simulink model "carModel"  (R2021a)
settings: Solver=ode15s  StartTime=0.0  StopTime=50  MaxStep=0.5  RelTol=1e-3
values from neighbouring files (symbols this model uses):
  initialFuel = 100    [data.m]
  maxEngineTemp = 240    [data.m]
  maxEngineTorque = 80    [data.m]
  maxMotorTemp = 135    [data.m]
  maxMotorTorque = 80    [data.m]
  maxRegenTorque = 80    [data.m]
  motorVoltage = 140    [data.m]
undefined symbols (not defined in the file or in its folder): b, k, Lock, N, sigbuilder_block, Temp_bpts, up
libraries: autolibsharedcoupling x7, autolibshared x7, autolibpowerinfoutils x4, autolibshareddiff x3, autolibhevctrlrcommon x2, autolibtrqconv x2, autolibutils x2, autolibtransamt x1, autolibsharedtransfixedgear x1, autolibdcdc x1, autolibdatasheetbattery x1, autolibmappedmotor x1
(part 1 of 6)
settings Model: EnablePacing=on  PacingRate=10  Creator=peter  LastModifiedBy=peter
settings DebuggingCC: SFMachineParentedDataDiag=warning

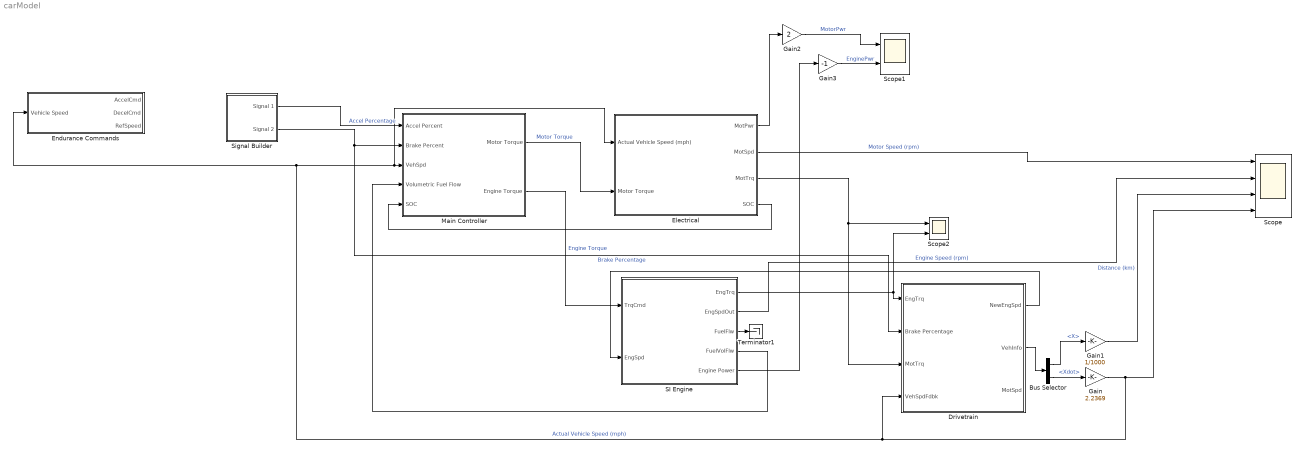
== system carModel ==
  Bus Selector : BusSelector  OutputSignals=InertFrm.Cg.Disp.X,InertFrm.Cg.Vel.Xdot
  Drivetrain : Subsystem
  Electrical : Subsystem
  Endurance Commands : Subsystem
  Gain : Gain  Gain=2.2369
  Gain1 : Gain  Gain=1/1000
  Gain2 : Gain  Gain=2
  Gain3 : Gain  Gain=-1
  Main Controller : Subsystem
  SI Engine : Subsystem
  Scope : Scope  NumInputPorts=4
  Scope1 : Scope  NumInputPorts=2
  Scope2 : Scope  NumInputPorts=2
  Signal Builder : Subsystem  Tag=STV Subsys  LoadFcn=sigbuilder_block('load');  StartFcn=sigbuilder_block('start');  StopFcn=sigbuilder_block('stop');  ClipboardFcn=sigbuilder_block('clipboard');  mask(Sigbuilder block){tuvar=[0:10]}
      mask help: Simulink:masks:SigbuilderBlock_MD
      mask init:
      | if ~strcmp(get_param(bdroot(gcbh),'SimulationStatus'),'stopped') tuvar = sigbuilder_block('maskInit'); end
      settings: CopyFcn=sigbuilder_block('copy');  DeleteFcn=sigbuilder_block('delete');  ModelCloseFcn=sigbuilder_block('modelClose');  PreSaveFcn=sigbuilder_block('preSave');  PauseFcn=sigbuilder_block('pause');  ContinueFcn=sigbuilder_block('continue');  NameChangeFcn=sigbuilder_block('namechange');  OpenFcn=sigbuilder_block('open',[1896 -18 550.8 400.2 ]);  CloseFcn=sigbuilder_block('close');
      mask Display: plot(0, 0, 100, 100,[2, 2, 32, 32, 2], [68, 8, 8, 68, 68],[32, 2], [38, 38], [32, 19, 2],[53, 60, 44], [32, 17, 17, 2],[16, 16, 31, 31]);txt = getActiveGroup(gcbh);text(2, 100, txt,'verticalAlignment', 'top');
  Terminator1 : Terminator
  wires:
  Electrical/4(SOC) -> Main Controller/5(SOC)
  Main Controller/1(Motor Torque) -> Electrical/2(Motor Torque)  "Motor Torque"
  Main Controller/2(Engine Torque) -> SI Engine/1(TrqCmd)  "Engine Torque"
  Drivetrain/1(NewEngSpd) -> SI Engine/2(EngSpd)
  SI Engine/3(FuelFlw) -> Terminator1/1
  SI Engine/4(FuelVolFlw) -> Main Controller/4(Volumetric Fuel Flow)
  SI Engine/1(EngTrq) -> Scope2/2, Drivetrain/1(EngTrq)
  Electrical/3(MotTrq) -> Drivetrain/3(MotTrq), Scope2/1
  Electrical/2(MotSpd) -> Scope/1  "Motor Speed (rpm)"
  Drivetrain/2(VehInfo) -> Bus Selector/1
  Bus Selector/1 -> Gain1/1  "<X>"
  Bus Selector/2 -> Gain/1  "<Xdot>"
  Gain/1 -> Scope/4, Drivetrain/4(VehSpdFdbk), Endurance Commands/1(Vehicle Speed), Electrical/1(Actual Vehicle Speed (mph)), Main Controller/3(VehSpd)  "Actual Vehicle Speed (mph)"
  Gain1/1 -> Scope/3  "Distance (km)"
  SI Engine/5(Engine Power) -> Gain3/1
  Electrical/1(MotPwr) -> Gain2/1
  Gain2/1 -> Scope1/1  "MotorPwr"
  Gain3/1 -> Scope1/2  "EnginePwr"
  SI Engine/2(EngSpdOut) -> Scope/2  "Engine Speed (rpm)"
  Signal Builder/1(Signal 1) -> Main Controller/1(Accel Percent)  "Accel Percentage"
  Signal Builder/2(Signal 2) -> Drivetrain/2(Brake Percentage), Main Controller/2(Brake Percent)  "Brake Percentage"

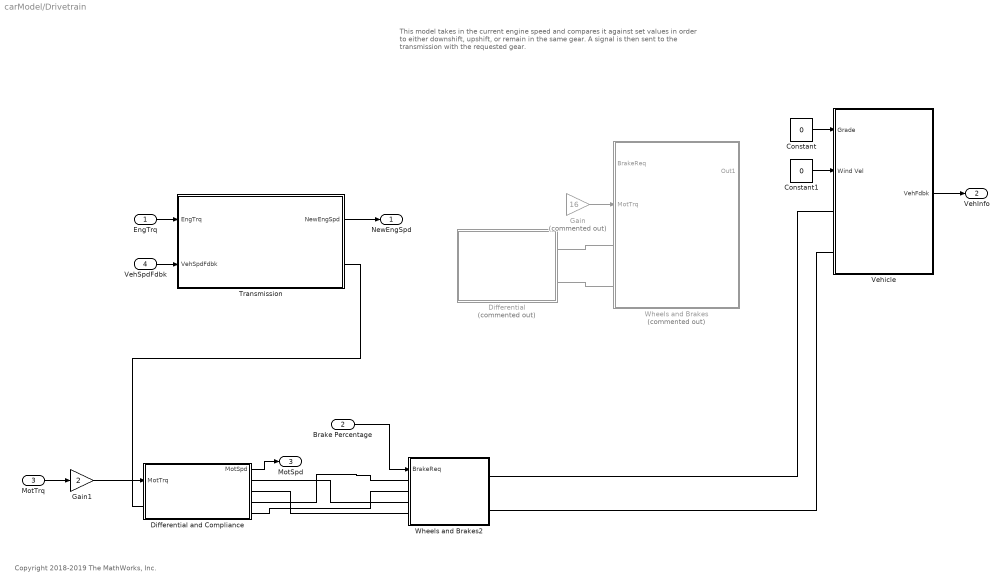
== system carModel/Drivetrain ==
  note: This model takes in the current engine speed and compares it against set values in order to either downshift, upshift, or remain in the same gear. A signal is then sent to the transmission with the requested gear.
  note: Copyright 2018-2019 The MathWorks, Inc.
  EngTrq : Inport
  Brake Percentage : Inport  Port=2
  MotTrq : Inport  Port=3
  VehSpdFdbk : Inport  Port=4
  Constant : Constant  Value=0
  Constant1 : Constant  Value=0
  Differential : Subsystem  Commented=on
  Differential and Compliance : Subsystem  VariantControl=2
  Gain : Gain  Commented=on  Gain=16
  Gain1 : Gain  Gain=2
  Transmission : Subsystem
  Vehicle : Subsystem
  Wheels and Brakes : Subsystem  Commented=on  VariantControl=0
  Wheels and Brakes2 : Subsystem  VariantControl=0
  NewEngSpd : Outport
  VehInfo : Outport  Port=2
  MotSpd : Outport  Port=3  VectorParamsAs1DForOutWhenUnconnected=off  BusOutputAsStruct=on
  wires:
  Constant/1 -> Vehicle/1(Grade)
  Constant1/1 -> Vehicle/2(Wind Vel)
  VehSpdFdbk/1 -> Transmission/2(VehSpdFdbk)
  Transmission/1(NewEngSpd) -> NewEngSpd/1
  Vehicle/1(VehFdbk) -> VehInfo/1
  Gain/1 -> Wheels and Brakes/2(MotTrq)
  EngTrq/1 -> Transmission/1(EngTrq)
  Differential and Compliance/1(MotSpd) -> MotSpd/1
  MotTrq/1 -> Gain1/1
  Brake Percentage/1 -> Wheels and Brakes2/1(BrakeReq)
  Gain1/1 -> Differential and Compliance/1(MotTrq)
  connections:
  Differential/RConn1 -- Wheels and Brakes/LConn1
  Differential/RConn2 -- Wheels and Brakes/LConn2
  Wheels and Brakes2/RConn2 -- Vehicle/LConn2
  Wheels and Brakes2/RConn1 -- Vehicle/LConn1
  Transmission/RConn1 -- Differential and Compliance/LConn1
  Differential and Compliance/RConn1 -- Wheels and Brakes2/LConn3
  Differential and Compliance/RConn2 -- Wheels and Brakes2/LConn4
  Differential and Compliance/RConn3 -- Wheels and Brakes2/LConn1
  Differential and Compliance/RConn4 -- Wheels and Brakes2/LConn2

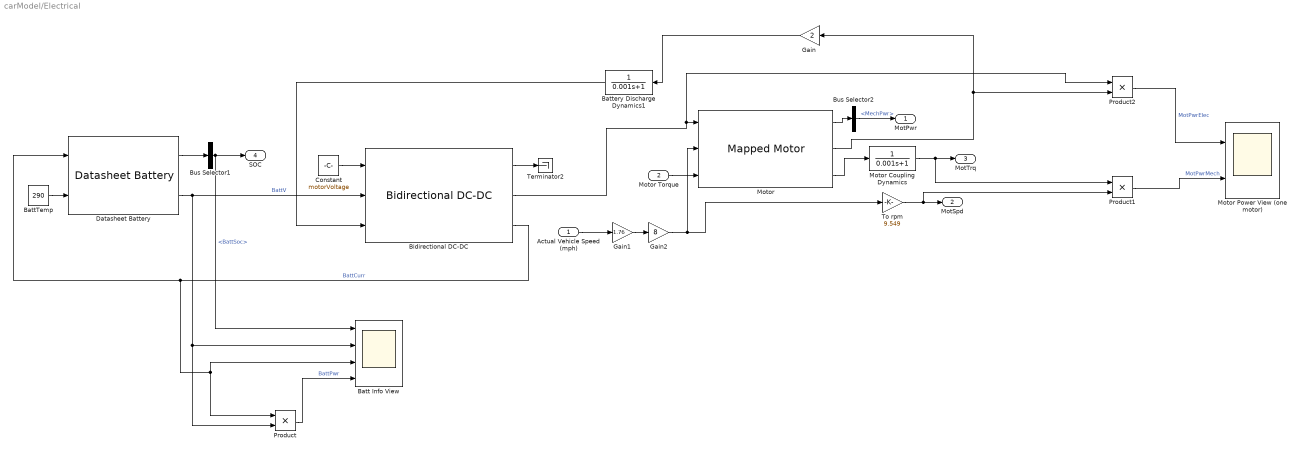
== system carModel/Electrical ==
  Actual Vehicle Speed (mph) : Inport
  Motor Torque : Inport  Port=2
  Batt Info View : Scope  NumInputPorts=4
  BattTemp : Constant  Value=290
  Battery Discharge Dynamics1 : TransferFcn  Denominator=[0.001 1]
  Bidirectional DC-DC : autolibdcdc/Bidirectional DC-DC  Tc=1/1000  Vinit=motorVoltage  Plimit=30000  param_loss=Single efficiency measurement  eff=98  v_loss_bp=[0 200 400 600 800 1000]  i_loss_bp=[0 25 50 75 100]  losses_table=[100 100 100 100 100;100 150 200 250 300;100 200 300 400 500;100 250 400 550 700;100 300 500 700 900;100 350 600 850 1100]  v_eff_bp=[200 400 600 800 1000]  i_eff_bp=[25 50 75 100]  efficiency_table=[96.2 98.1 98.7 99;98.1 99 99.4 99.5;98.7 99.4 99.6 99.7;99 99.5 99.7 99.8;99.2 99.6 99.7 99.8]  x_v_bp=[-1000 -800 -600 -400 -200 200 400 600 800 1000]  x_i_bp=[-100 -75 -50 -25 25 50 75 100]  x_losses_mat=[200.400801603196 225.67703109328 200.803212851408 201.612903225806 199.999999999997 200 225 200;160.320641282556 180.541624874624 201.005025125625 202.020202020203 200 200 180 160;180.541624874624 180.722891566267 181.086519114686 197.568389057748 194.999999999999 179.999999999997 180 180;201.005025125625 181.086519114686 202.020202020203 193.67991845056 190 200 179.999999999997 200;202.020202020203 197.568389057748 193.67991845056 197.505197505197 190 190 194.999999999999 200;200 194.999999999999 190 190 197.505197505197 193.67991845056 197.568389057748 202.020202020203;200 179.999999999997 200 190 193.67991845056 202.020202020203 181.086519114686 201.005025125625;180 180 179.999999999997 194.999999999999 197.568389057748 181.086519114686 180.722891566267 180.541624874624;160 180 200 200 202.020202020203 201.005025125625 180.541624874624 160.320641282556;200 225 200 199.999999999997 201.612903225806 200.803212851408 225.67703109328 200.400801603196]  RefBlkName='autolibdcdc/Bidirectional DC-DC'
      settings: SourceProductBaseCode=PW
  Bus Selector1 : BusSelector  OutputSignals=BattSoc
  Bus Selector2 : BusSelector  OutputSignals=MechPwr
  Constant : Constant  Value=motorVoltage
  Datasheet Battery : autolibdatasheetbattery/Datasheet Battery  CapacityCtrl=Parameter  OutputVlt=Filtered  BattChargeMax=2.5  Em=[2.8 3.228 3.284 3.361 3.408 3.427 3.472 3.477 3.493 3.504 3.516 3.528 3.537 3.545 3.555 3.561 3.566 3.576 3.587 3.589 3.594 3.6 3.608 3.61 3.616 3.619 3.626 3.632 3.637 3.64 3.645 3.646 3.652 3.655 3.658 3.661 3.664 3.668 3.673 3.678 3.68 3.681 3.686 3.692 3.699 3.702 3.705 3.71 3.717 3.723 3.728 3.733 3.735 3.742 3.749 3.755 3.761 3.768 3.773 3.78 3.791 3.798 3.798 3.814 3.818 3.825 3.841 3.846 3.855 3.863 3.877 3.885 3.894 3.907 3.919 3.926 3.935 3.944 3.954 3.964 3.974 3.988 3.998 4.014 4.029 4.034 4.047 4.065 4.074 4.086 4.097 4.131 4.126 4.138 4.15 4.18 4.174 4.187 4.207 4.231 4.221]  CapLUTBp=[0 0.01 0.02 0.03 0.04 0.05 0.06 0.07 0.08 0.09 0.1 0.11 0.12 0.13 0.14 0.15 0.16 0.17 0.18 0.19 0.2 0.21 0.22 0.23 0.24 0.25 0.26 0.27 0.28 0.29 0.3 0.31 0.32 0.33 0.34 0.35 0.36 0.37 0.38 0.39 0.4 0.41 0.42 0.43 0.44 0.45 0.46 0.47 0.48 0.49 0.5 0.51 0.52 0.53 0.54 0.55 0.56 0.57 0.58 0.59 0.6 0.61 0.62 0.63 0.64 0.65 0.66 0.67 0.68 0.69 0.7 0.71 0.72 0.73 0.74 0.75 0.76 0.77 0.78 0.79 0.8 0.81 0.82 0.83 0.84 0.85 0.86 0.87 0.88 0.89 0.9 0.91 0.92 0.93 0.94 0.95 0.96 0.97 0.98 0.99 1]  RInt=[0.008846 0.009319 0.009027 0.00847 0.01032 0.01314;0.006389 0.006554 0.005553 0.005525 0.006043 0.007805;0.004364 0.004101 0.00406 0.003452 0.003846 0.004517;0.002031 0.002563 0.002532 0.00246 0.002716 0.003047;0.001443 0.001825 0.001795 0.001778 0.001924 0.002234;0.0005603 0.0007192 0.0006887 0.0007557 0.0007355 0.001014;0.001028 0.001338 0.001 0.001536 0.001546 0.002789]  BattTempBp=[243.1 253.1 263.1 273.1 283.1 298.1 313.1]  CapSOCBp=[0 0.2 0.4 0.6 0.8 1]  Ns=32  Np=9  BattCapInit=2.5  Tc=1/1000  Vinit=4.221  RefBlkName='autolibdatasheetbattery/Datasheet Battery'
      settings: SourceProductBaseCode=PW
  Gain : Gain  Gain=2
  Gain1 : Gain  Gain=1.76
  Gain2 : Gain  Gain=8
  Motor : autolibmappedmotor/Mapped Motor  port_config=Speed  param_by=Tabulated torque-speed envelope  w_t=motorSpeeds  T_t=motorTorques  torque_max=80  power_max=30000  Tc=0.02  param_loss=Tabulated efficiency data  eff=88  w_eff=419  T_eff=26  Piron=0  Pbase=0  w_eff_bp=motorSpeeds  T_eff_bp=efficiencyTrq  Temp_eff_bp=[233.15 293.15 373.15]  losses_table=[1.49 1.67 2.21 3.10; 0.42 0.69 1.14 2.03; 0.06 0.24 0.78 1.68; 0.42 0.69 1.14 2.03; 1.49 1.67 2.21 3.10]  losses_table_3d=cat(3,1.05*[1.49 1.67 2.21 3.10; 0.42 0.69 1.14 2.03; 0.06 0.24 0.78 1.68; 0.42 0.69 1.14 2.03; 1.49 1.67 2.21 3.10],[1.49 1.67 2.21 3.10; 0.42 0.69 1.14 2.03; 0.06 0.24 0.78 1.68; 0.42 0.69 1.14 2.03; 1.49 1.67 2.21 3.10],1.03*[1.49 1.67 2.21 3.10; 0.42 0.69 1.14 2.03; 0.06 0.24 0.78 1.68; 0.42 0.69 1.14 2.03; 1.49 1.67 2.21 3.10])  efficiency_table=efficiency  efficiency_table_3d=cat(3,90*ones(5,4),95*ones(5,4),92*ones(5,4))  J=.042  b=1e-5  omega_o=0  T_t_extended=[40.93 44.07 47.75 52.09 57.3 63.66 71.62 80 80 80 80 80 80 80 80 80 80 80 80 80 80 80 71.62 63.66 57.3 52.09 47.75 44.07 40.93]  w_t_extended=[-733.038285837618 -680.678408277789 -628.318530717959 -575.958653158129 -523.598775598299 -471.238898038469 -418.879020478639 -374.999123017327 -314.159265358979 -261.799387799149 -209.43951023932 -157.07963267949 -104.71975511966 -52.3598775598299 0 52.3598775598299 104.71975511966 157.07963267949 209.43951023932 261.799387799149 314.159265358979 374.999123017327 418.879020478639 471.238898038469 523.598775598299 575.958653158129 628.318530717959 680.678408277789 733.038285837618]  KLossIron=0  KLossCopper=2.1976  x_w_eff_vec=[-733.038285837618 -680.678408277789 -628.318530717959 -575.958653158129 -523.598775598299 -471.238898038469 -418.879020478639 -374.999123017327 -314.159265358979 -261.799387799149 -209.43951023932 -157.07963267949 -104.71975511966 -52.3598775598299 0 52.3598775598299 104.71975511966 157.07963267949 209.43951023932 261.799387799149 314.159265358979 374.999123017327 418.879020478639 471.238898038469 523.598775598299 575.958653158129 628.318530717959 680.678408277789 733.038285837618]  x_T_eff_vec=[-79.996 -74.282 -68.568 -62.854 -57.14 -51.426 -45.712 -39.998 -34.284 -28.57 -22.856 -17.142 -11.428 -5.714 0 5.714 11.428 17.142 22.856 28.57 34.284 39.998 45.712 51.426 57.14 62.854 68.568 74.282 79.996]  x_tmp_eff_vec=[233.15 293.15 373.15]  x_losses_mat=[4413.77327953831 4098.50375957128 3783.23423960426 3467.96471963724 3152.69519967022 2837.4256797032 2522.15615973618 2206.88663976915 1891.61711980213 1576.34759983511 1261.07807986809 945.808559901066 828.510481043633 681.861985044955 0 586.401307138661 753.944537749707 879.601960707991 1172.80261427732 1466.00326784665 1759.20392141598 2052.40457498531 2345.60522855464 2638.80588212397 2932.0065356933 3225.20718926263 3518.40784283196 3811.6084964013 4104.80914997063;4098.50375957128 3805.75349103048 3513.00322248967 3220.25295394887 2927.50268540806 2634.75241686725 2342.00214832645 2049.25187978564 1756.50161124484 1463.75134270403 1171.00107416322 878.250805622418 769.331160969088 633.157557541744 0 544.5154994859 700.091356481871 816.773249228849 1089.0309989718 1361.28874871475 1633.5464984577 1905.80424820065 2178.0619979436 2450.31974768655 2722.5774974295 2994.83524717245 3267.0929969154 3539.35074665835 3811.6084964013;3783.23423960426 3513.00322248967 3242.77220537508 2972.54118826049 2702.3101711459 2432.07915403131 2161.84813691672 1891.61711980213 1621.38610268754 1351.15508557295 1080.92406845836 810.693051343771 624.384710351724 584.453130038533 0 502.629691833138 574.433933523586 753.944537749707 1005.25938366628 1256.57422958284 1507.88907549941 1759.20392141598 2010.51876733255 2261.83361324912 2513.14845916569 2764.46330508226 3015.77815099883 3267.0929969154 3518.40784283197;3467.96471963724 3220.25295394887 2972.54118826049 2724.82942257212 2477.11765688374 2229.40589119537 1981.69412550699 1733.98235981862 1486.27059413025 1238.55882844187 990.847062753497 743.135297065123 572.352651155747 535.748702535322 0 460.743884180377 526.564439063287 691.115826270564 921.487768360753 1151.85971045094 1382.23165254113 1612.60359463132 1842.97553672151 2073.34747881169 2303.71942090188 2534.09136299207 2764.46330508226 2994.83524717245 3225.20718926263;3152.69519967022 2927.50268540806 2702.3101711459 2477.11765688374 2251.92514262159 2026.73262835943 1801.54011409727 1576.34759983511 1351.15508557295 1125.96257131079 900.770057048634 675.577542786476 591.793200745452 487.044275032111 0 418.858076527615 538.531812678362 628.287114791422 837.71615305523 1047.14519131904 1256.57422958284 1466.00326784665 1675.43230611046 1884.86134437427 2094.29038263807 2303.71942090188 2513.14845916569 2722.5774974295 2932.0065356933;2837.4256797032 2634.75241686725 2432.07915403131 2229.40589119537 2026.73262835943 1824.05936552348 1621.38610268754 1418.7128398516 1216.03957701566 1013.36631417971 810.693051343771 608.019788507828 532.613880670907 438.3398475289 0 376.972268874854 484.678631410526 565.45840331228 753.944537749707 942.430672187133 1130.91680662456 1319.40294106199 1507.88907549941 1696.37520993684 1884.86134437427 2073.34747881169 2261.83361324912 2450.31974768655 2638.80588212397;2522.15615973618 2342.00214832645 2161.84813691672 1981.69412550699 1801.54011409727 1621.38610268754 1441.23209127781 1261.07807986809 1080.92406845836 900.770057048634 832.512947135632 624.384710351724 531.883271781099 455.899947240942 0 382.955955682391 478.694944602989 574.433933523586 765.911911364782 837.71615305523 1005.25938366628 1172.80261427732 1340.34584488837 1507.88907549941 1675.43230611046 1842.97553672151 2010.51876733255 2178.0619979436 2345.60522855464;2257.94633241138 2096.66445152485 1935.38257063833 1774.1006897518 1612.81880886527 1451.53692797875 1290.25504709222 1128.97316620569 967.691285319163 931.628256052611 847.679336276441 635.759502207331 584.384996978457 470.358656104611 0 385.694098005781 514.258797341042 578.541147008672 771.388196011562 857.097995568402 899.952895346822 1049.94504457129 1199.93719379576 1349.92934302023 1499.9214922447 1649.91364146917 1799.90579069364 1949.89793991811 2099.89008914258;2485.5314431309 2307.99348290726 1873.15413105517 1717.05795346724 1560.96177587931 1404.86559829138 1248.76942070345 1092.67324311552 936.577065527586 887.689801118178 710.151840894543 ...(+9364 chars)]  x_losses_mat_3d=cat(3,[3.255 2.3205 1.7535 1.5645 1.7535 2.3205 3.255;2.1315 1.197 0.7245 0.441 0.7245 1.197 2.1315;1.764 0.819 0.252 0.063 0.252 0.819 1.764;2.1315 1.197 0.7245 0.441 0.7245 1.197 2.1315;3.255 2.3205 1.7535 1.5645 1.7535 2.3205 3.255],[3.1 2.21 1.67 1.49 1.67 2.21 3.1;2.03 1.14 0.69 0.42 0.69 1.14 2.03;1.68 0.78 0.24 0.06 0.24 0.78 1.68;2.03 1.14 0.69 0.42 0.69 1.14 2.03;3.1 2.21 1.67 1.49 1.67 2.21 3.1],[3.193 2.2763 1.7201 1.5347 1.7201 2.2763 3.193;2.0909 1.1742 0.7107 0.4326 0.7107 1.1742 2.0909;1.7304 0.8034 0.2472 0.0618 0.2472 0.8034 1.7304;2.0909 1.1742 0.7107 0.4326 0.7107 1.1742 2.0909;3.193 2.2763 1.7201 1.5347 1.7201 2.2763 3.193])  CalLossMapData={}  CalLossWithTempMapData={}  aMode=2  RefBlkName='autolibmappedmotor/Mapped Motor'
      settings: SourceProductBaseCode=PW,DR,MT,UV,VE
  Motor Coupling Dynamics : TransferFcn  Denominator=[0.001 1]
  Motor Power View (one motor) : Scope  NumInputPorts=2
  Product : Product
  Product1 : Product
  Product2 : Product
  Terminator2 : Terminator
  To rpm : Gain  Gain=9.549
  MotPwr : Outport
  MotSpd : Outport  Port=2
  MotTrq : Outport  Port=3
  SOC : Outport  Port=4
  wires:
  BattTemp/1 -> Datasheet Battery/2
  Datasheet Battery/1 -> Bus Selector1/1
  Motor/2 -> Gain/1, Product2/2
  Bus Selector1/1 -> Batt Info View/1, SOC/1  "<BattSoc>"
  Motor/1 -> Bus Selector2/1
  Motor Torque/1 -> Motor/3
  Motor/3 -> Motor Coupling Dynamics/1
  Motor Coupling Dynamics/1 -> Product1/1, MotTrq/1
  Bidirectional DC-DC/2 -> Product2/1, Motor/1
  Datasheet Battery/2 -> Bidirectional DC-DC/2, Product/2, Batt Info View/2  "BattV"
  Constant/1 -> Bidirectional DC-DC/1
  Bidirectional DC-DC/3 -> Product/1, Batt Info View/3, Datasheet Battery/1  "BattCurr"
  Battery Discharge Dynamics1/1 -> Bidirectional DC-DC/3
  Bidirectional DC-DC/1 -> Terminator2/1
  To rpm/1 -> Product1/2, MotSpd/1
  Product/1 -> Batt Info View/4  "BattPwr"
  Product1/1 -> Motor Power View (one motor)/2  "MotPwrMech"
  Product2/1 -> Motor Power View (one motor)/1  "MotPwrElec"
  Bus Selector2/1 -> MotPwr/1  "<MechPwr>"
  Gain/1 -> Battery Discharge Dynamics1/1
  Gain1/1 -> Gain2/1
  Actual Vehicle Speed (mph)/1 -> Gain1/1
  Gain2/1 -> To rpm/1, Motor/2

== system carModel/Endurance Commands ==
  Vehicle Speed : Inport
  Constant : Constant  Value=0
  Drive Cycle Source : autolibshared/Drive Cycle Source  cycleVar=FTP75  fileVar=cycleFTP75.mat  tfinal="2474  seconds"  cycleRepeat=off  outAccPort=off  outGearPort=off  gearList=No gear data  t_wot1=5  xdot_woto=0  xdot_wot1=30  t_wot2=20  xdot_wot2=0  t_wotend=30  srcUnit=m/s  outUnit=mph  srcAccUnit=m/s/s  outAccUnit=m/s^2  dt=0  aMode=2  faultOption=off  velBnd=2  velBndUnit=mph  inUnit=m/s  timeBnd=1  failOption=off  stopSim=off  maxFaultCnt=10  maxFaultTime=2  maxTotFaultTime=15  traceOption=off  dtTrace=1  traceWindow=10  lastDCname=FTP75  lastOutUnit=mph  lastDT=0  lastTB=1  lastSB=2  forceCalcBound=off
      settings: SourceProductBaseCode=PW,DR,MT,UV,VE
  Gain : Gain  Gain=1.75
  Longitudinal Driver : autolibshared/Longitudinal Driver  extAccelOvr=off  extDecelOvr=off  extAccelHld=off  extDecelHld=off  extAccelZero=off  extDecelZero=off  cntrlType=PI  shftType=None  velUnits=mph  gearOut=off  Kp=10  Ki=5  Kff=.1  Kg=0  VehVelVec=[0 100]  KffVec=[.1 .1]  KpVec=[10 10]  KiVec=[5 5]  KgVec=[0 0]  m=1500  Kpt=3000  tau=.1  L=2  aR=200  bR=2.5  cR=.5  g=9.81  vnom=5  Kaw=1  tauerr=.01  tauPt=2  GearInit=0  tShift=.1  pdlVec=[0.1 0.4 0.5 0.9]  upShftTbl=[-1 12.9375 26.4375 39.9375 51.18749999999999 62.4375 72.84375 83.25;-1 16.3125 29.8125 43.3125 54.5624 65.8125 76.78125 87.75;-1 19.6875 33.1875 46.68749999999999 57.9375 69.1875 80.71875 92.25;-1 33 52.5 77.25 100.5 138.75 161.875 185]  dwnShftTbl=[1 9.5625 23.0625 36.5625 47.8125 59.0625 68.90625 78.75;1 12.9375 26.4375 39.9375 51.18749999999999 62.4375 72.84375 83.25;1 16.3125 29.8125 43.3125 54.562499 65.8125 76.78125 87.75;1 19.6875 33.1875 46.68749999999999 57.9375 69.1875 80.71875 92.25]  tClutch=.5  tRev=.5  tPark=120  aMode=2  UpGearVec="[0  1  2  3  4  5  6  7]"  DownGearVec="[1  2  3  4  5  6  7  8]"
      settings: SourceProductBaseCode=PW,DR,MT,UV,VE
  Terminator4 : Terminator
  AccelCmd : Outport
  DecelCmd : Outport  Port=2
  RefSpeed : Outport  Port=3
  wires:
  Vehicle Speed/1 -> Longitudinal Driver/2
  Constant/1 -> Longitudinal Driver/3
  Drive Cycle Source/1 -> Gain/1
  Longitudinal Driver/2 -> AccelCmd/1
  Longitudinal Driver/1 -> Terminator4/1
  Longitudinal Driver/3 -> DecelCmd/1
  Gain/1 -> RefSpeed/1, Longitudinal Driver/1

== system carModel/Main Controller ==
  Accel Percent : Inport
  Brake Percent : Inport  Port=2
  VehSpd : Inport  Port=3
  Volumetric Fuel Flow : Inport  Port=4
  SOC : Inport  Port=5
  Fuel and SOC Checks : Subsystem
  Heat Controller : Subsystem
  Optimizes torques for best efficiency : Subsystem
  Scope : Scope  NumInputPorts=2
  Sets torques to their final values : Subsystem
  Motor Torque : Outport
  Engine Torque : Outport  Port=2
  wires:
  Accel Percent/1 -> Sets torques to their final values/7(Accel Percent), Optimizes torques for best efficiency/2(Accelerator Value)
  VehSpd/1 -> Optimizes torques for best efficiency/1(Speed), Fuel and SOC Checks/1(VehSpd)
  Volumetric Fuel Flow/1 -> Fuel and SOC Checks/2(Volumetric Fuel Flow)
  SOC/1 -> Fuel and SOC Checks/3(SOC)
  Heat Controller/1(Updated Motor Torque) -> Scope/1, Motor Torque/1  "MotTrq"
  Heat Controller/2(Updated Engine Torque) -> Scope/2, Engine Torque/1  "EngTrq"
  Optimizes torques for best efficiency/1(Initial Engine Torque) -> Sets torques to their final values/1(Initial Engine Torque)
  Optimizes torques for best efficiency/2(Initial Motor Torque) -> Sets torques to their final values/2(Initial Motor Torque)
  Fuel and SOC Checks/1(MaxMotTrq) -> Sets torques to their final values/3(MaxMotTrq)
  Fuel and SOC Checks/2(MaxEngTrq) -> Sets torques to their final values/4(MaxEngTrq)
  Fuel and SOC Checks/3(MaxRegenTrq) -> Sets torques to their final values/5(MaxRegenTrq)
  Brake Percent/1 -> Sets torques to their final values/6(Brake Percent)
  Sets torques to their final values/1(MotTrq) -> Heat Controller/1(Motor Torque)
  Sets torques to their final values/2(EngTrq) -> Heat Controller/2(Engine Torque)
